simulink model "PMSM_ADRC_position_V21"  (R2024b)
settings: Solver=ode3  StartTime=0.0  StopTime=0.5  FixedStep=1e-6  RelTol=1e-3
model workspace (MAT data in the model file):
  PWM_Frequency = Simulink.Parameter
  PWM_Frequency.Value = 72000
  PWM_Frequency.Complexity = 'real'
  PWM_Frequency.Dimensions = [1 1]
  PWM_Frequency.DataType = 'double'
  TimerPeriod = 0.1
  Vdc = 12
  b0_id = 1333.33333333
  b0_iq = 1000
  b0_pos = 500
  idiq_ctrl_freq = 8000
  kd_pos = 200
  kp_id = 800
  kp_iq = 800
  kp_pos = 10000
  pos_ctrl_freq = 2000
  wc_pos = 50
  wo_id = 2000
  wo_iq = 2000
  wo_pos = 1000
undefined symbols (not defined in the file): Down, Up
libraries: eePwmGenerator x5, spsDCVoltageSourceLib x1, spsPermanentMagnetSynchronousMachineLib x1, spsUniversalBridgeLib x1, spspowerguiLib x1
settings Model: ParameterArgumentNames=wc_pos  Creator=shish  LastModifiedBy=HZSK

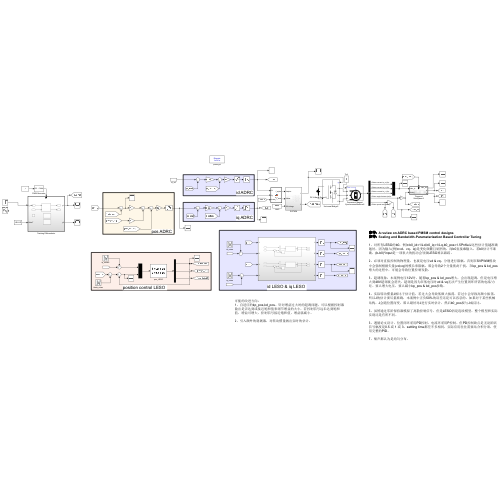
[thumbnail: Simulink's stored preview of the top-level diagram]
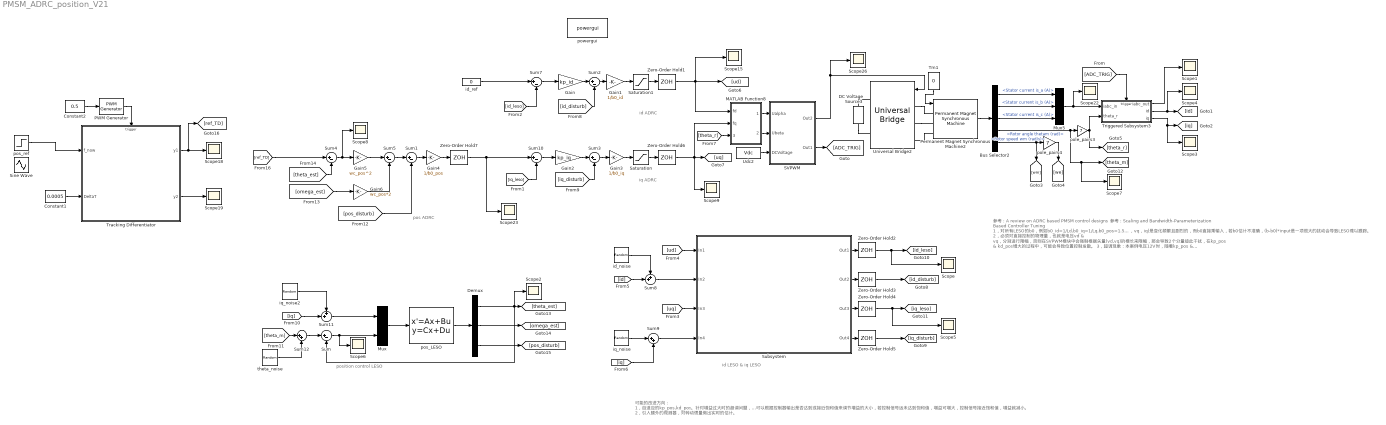
== system PMSM_ADRC_position_V21 ==
  note: 可能的改进方向：
      | 1，自适应的kp_pos,kd_pos。针对增益过大时的超调问题，可以根据控制器输出是否达到或接近饱和值来调节增益的大小，若控制信号远未达到饱和值，增益可增大，控制信号接近饱和值，增益就减小。
      |
      | 2，引入额外的观测器，对转动惯量做出实时的估计。
  note: id LESO & iq LESO
  note: 参考：A review on ADRC based PMSM control designs
      | 参考：Scaling and Bandwidth-Parameterization Based Controller Tuning
      |
      | 1，对所有LESO的b0，例如b0_id=1/Ld,b0_iq=1/Lq,b0_pos=1.5PnKe/J这些估计值越准确越好，因为输入(例如vd，vq，iq)是变化频繁且剧烈的，而b0直接乘输入，若b0估计不准确，(b-b0)*input是一项很大的扰动会导致LESO难以跟踪。
      |
      | 2，必须对直接控制的物理量，也就是电压vd & vq，分别进行限幅，否则在SVPWM模块中会强制根据矢量(vd,vq)的模长来限幅，那会导致2个分量彼此干扰，在kp_pos & kd_pos增大的过程中，可能会导致位置控制发散。
      |
      | 3，超调现象：本案例电压12V时，随着kp_pos & kd_pos增大，会出现超调，但是电压增大到48V超调就会消失。超调是因为在低电压时vd & vq无法产生位置闭环所需的电流/力矩。要么增大电压，要么减小kp_pos & kd_pos参数。
      |
      | 4，实际转动惯量J相比于估计值，若过大会导致低频大振荡，若过小会导致高频小振荡。所以J的估计要尽量准确，本案例中正负50%的误差还是可以容忍的。如果对于某些机械结构，J会随位置而变，那么最好对J进行实时估计，然后b0_pos要与J成反比。
      |
      | 5，虽然通过零阶保持器模拟了离散控制信号，但是LESO仍是连续模型，整个模型和实际实现还是有所不同。
      |
      | 6，遵循论文设计，位置闭环采用PD控制，电流环采用P控制。但PD控制缺点是无论阶跃信号幅度是0.5 或 1 或 3，settling time都差不多相同，实际应用往往需要结合积分项，使用完整的PID。
      |
      | 7，噪声都认为是均匀分布。
  note: position control LESO
  note: pos ADRC
  note: iq ADRC
  note: id ADRC
  Bus Selector2 : BusSelector  OutputSignals=Stator current is_a (A),Stator current is_b (A),Stator current is_c (A),Rotor angle thetam (rad),Rotor speed wm (rad/s)
  Constant1 : Constant  Value=0.0005
  Constant2 : Constant  Value=0.5
  DC Voltage Source3 : spsDCVoltageSourceLib/DC Voltage Source  Amplitude=Vdc  Measurements=Voltage
  Demux : Demux  Outputs=3
  Gain : Gain  Gain=kp_id
  Gain1 : Gain  Gain=1/b0_id
  Gain2 : Gain  Gain=kp_iq
  Gain3 : Gain  Gain=1/b0_iq
  Gain4 : Gain  Gain=1/b0_pos
  Gain5 : Gain  Gain=wc_pos^2
  Gain6 : Gain  Gain=wc_pos*2
  MATLAB Function8 : MATLAB Function  TreatAsAtomicUnit=on
  Mux : Mux  Inputs=2
  Mux5 : Mux  Inputs=3
  PWM Generator : eePwmGenerator/PWM Generator  CarrCount=Up  Tper=0.0005  Tdelay=0  Ts=5e-5
  Permanent Magnet Synchronous Machine2 : spsPermanentMagnetSynchronousMachineLib/Permanent Magnet Synchronous Machine  NbPhases=3  FluxDistribution=Sinusoidal  RotorType=Salient-pole  MechanicalLoad=Torque Tm  PresetModel=No  ShowDetailedParameters=on  MeasurementBus=off  Resistance=3  Inductance=8.5e-3  dqInductances=[0.75e-3,1.0e-3]  La=0.000395  MachineConstant=Flux linkage established by magnets (V.s)  Flux=0.0012  VoltageCst=1.5236  TorqueCst=0.0126  Flat=120  Mechanical=[1.2e-5 5e-6 7 0]  PolePairs=4  InitialConditions=[0,0, 0,0]  InitialConditions5ph=[0 0 0 0 0 0]  RefAngle=Aligned with phase A axis (original Park)  IterativeDiscreteModel=Trapezoidal non iterative  TsBlock=-1  TsPowergui=0
  SVPWM : Subsystem
  Saturation : Saturate  UpperLimit=2*Vdc/3  LowerLimit=-2*Vdc/3
  Saturation1 : Saturate  UpperLimit=2*Vdc/3  LowerLimit=-2*Vdc/3
  Scope{,1..9,15,18..19,22..23,26} (16 alike) : Scope
  Sine Wave : Sin  Amplitude=2  Frequency=2*pi  SampleTime=0
  Subsystem : Subsystem
  Sum{,1..5,7,10} (8 alike) : Sum  Inputs=|+-
  Sum11 : Sum  Inputs=++|
  Sum12 : Sum  Inputs=|++
  Sum8 : Sum  Inputs=++|
  Sum9 : Sum  Inputs=|++
  Tm1 : Constant  Value=0
  Tracking Differentiator : Subsystem
  Triggered Subsystem3 : Subsystem  TreatAsAtomicUnit=on
  Udc2 : Constant  Value=Vdc
  Universal Bridge2 : spsUniversalBridgeLib/Universal Bridge  Arms=3  SnubberResistance=1e5  SnubberCapacitance=inf  Device=MOSFET / Diodes  Ron=1e-3  Lon=0  ForwardVoltages="[  0  0  ]"  ForwardVoltage=0  GTOparameters=[ 10e-6 , 20e-6 ]  IGBTparameters=[ 1e-6 , 2e-6 ]  Measurements=None  Measurements_2=None  converterType=Rectifier
  Zero-Order Hold{1..6} (6 alike) : ZeroOrderHold  SampleTime=1.0/idiq_ctrl_freq
  Zero-Order Hold7 : ZeroOrderHold  SampleTime=1.0/pos_ctrl_freq
  id_noise : UniformRandomNumber  Minimum=-0.005  Maximum=0.005  SampleTime=1.0/40000
  id_ref : Constant  Value=0
  iq_noise : UniformRandomNumber  Minimum=-0.005  Maximum=0.005  SampleTime=1.0/40000
  iq_noise2 : UniformRandomNumber  Minimum=-0.005  Maximum=0.005  SampleTime=1.0/40000
  pole_pairs3 : Gain  Gain=7
  pole_pairs4 : Gain  Gain=7
  pos_LESO : StateSpace  A=[0 1 0; 0 0 1; 0 0 0]  B=[0 3*wo_pos;b0_pos 3*wo_pos^2;0 wo_pos^3]  C=[1 0 0;0 1 0;0 0 1]  D=[0 0;0 0;0 0]  InitialCondition=0
  pos_ref : Step  Time=0.1  After=3.0  SampleTime=0
  powergui : spspowerguiLib/powergui  Priority=1  SimulationMode=Discrete  SampleTime=1e-6  frequency=60  Iterations=50  frequencyindice=0  Pbase=100e6  ErrMax=1e-4  UnitsV=kV  UnitsW=MW  buscounter=0  FunctionMessages=off  echomessages=off  EnableUseOfTLC=off  CurrentSourceSwitches=off  DisableSnubberDevices=off  DisableRonSwitches=off  DisableVfSwitches=off  DisplayEquations=off  AutomaticDiscreteSolvers=off  SolverType=Tustin/Backward Euler (TBE)  Interpol=off  ExternalGateDelay=off  methode=off  Ts=100  x0status=blocks  SPID=on  SwTol=0  HookPort=off  NonlinearTolerance=1e-4  nMaxIteration=100  ContinueOnMaxIteration=off  RestoreLinks=warning  ResistiveCurrentMeasurement=off  Frange=[0:2:500]  Ylog=off  Xlog=on  ShowGrid=off  save=off  variable=ZData  structure=0  ZoomFFT=off  StartTime=0.0  cycles=1  DisplayStyle=1  fundamental=60  FreqAxis=off  MaxFrequency=1000  frequencyindicesteady=1  RmsSteady=1  display=off
  theta_noise : UniformRandomNumber  Minimum=-0.5*2*pi/4096  Maximum=0.5*2*pi/4096  SampleTime=1.0/2000
  wires:
  Bus Selector2/5 -> pole_pairs4/1, [wm]  "<Rotor speed wm (rad/s)>"
  MATLAB Function8/2(f_beta) -> SVPWM/2(Ubeta)
  Bus Selector2/3 -> Mux5/3  "<Stator current is_c (A)>"
  MATLAB Function8/1(f_alpha) -> SVPWM/1(Ualpha)
  Permanent Magnet Synchronous Machine2/1 -> Bus Selector2/1
  Bus Selector2/4 -> Scope7/1, [theta_m], pole_pairs3/1  "<Rotor angle thetam (rad)>"
  Udc2/1 -> SVPWM/3(DCVoltage)
  Bus Selector2/2 -> Mux5/2  "<Stator current is_b (A)>"
  Mux5/1 -> Triggered Subsystem3/1(iabc_in), Scope22/1
  Tm1/1 -> Permanent Magnet Synchronous Machine2/1
  SVPWM/1(Out2) -> Scope26/1, Universal Bridge2/1
  Bus Selector2/1 -> Mux5/1  "<Stator current is_a (A)>"
  Triggered Subsystem3/2(id) -> [id], Scope4/1
  Triggered Subsystem3/3(iq) -> [iq], Scope3/1
  pole_pairs4/1 -> [we]
  SVPWM/2(Out1) -> [ADC_TRIG]
  [ADC_TRIG] -> Triggered Subsystem3/Trigger
  pole_pairs3/1 -> Triggered Subsystem3/2(theta_r), [theta_r]
  [theta_r] -> MATLAB Function8/3(theta_r)
  Triggered Subsystem3/1(iabc_out) -> Scope1/1
  Subsystem/1(Out1) -> Zero-Order Hold2/1
  Subsystem/3(Out3) -> Zero-Order Hold4/1
  [ud] -> Subsystem/1(In1)
  [uq] -> Subsystem/3(In3)
  Subsystem/4(Out4) -> Zero-Order Hold5/1
  Mux/1 -> pos_LESO/1
  Sum/1 -> Scope6/1, Mux/2
  pos_LESO/1 -> Demux/1
  [pos_disturb] -> Sum1/2
  Sum1/1 -> Gain4/1
  Sum4/1 -> Scope8/1, Gain5/1
  Gain5/1 -> Sum5/1
  Gain6/1 -> Sum5/2
  Sum5/1 -> Sum1/1
  [theta_est] -> Sum4/2
  Gain4/1 -> Zero-Order Hold7/1
  Constant1/1 -> Tracking Differentiator/2(DeltaT)
  Tracking Differentiator/1(y1) -> [ref_TD], Scope18/1
  Constant2/1 -> PWM Generator/1
  PWM Generator/1 -> Tracking Differentiator/Trigger
  Tracking Differentiator/2(y2) -> Scope19/1
  [ref_TD] -> Sum4/1
  [omega_est] -> Gain6/1
  [id] -> Sum8/2
  [iq] -> Sum9/2
  id_noise/1 -> Sum8/1
  Sum8/1 -> Subsystem/2(In2)
  iq_noise/1 -> Sum9/1
  Sum9/1 -> Subsystem/4(In4)
  [iq] -> Sum11/2
  Sum11/1 -> Mux/1
  Sum12/1 -> Sum/1
  [theta_m] -> Sum12/1
  theta_noise/1 -> Sum12/2
  iq_noise2/1 -> Sum11/1
  Saturation1/1 -> Zero-Order Hold1/1
  Sum3/1 -> Gain3/1
  Sum10/1 -> Gain2/1
  Zero-Order Hold7/1 -> Scope23/1, Sum10/1
  Gain3/1 -> Saturation/1
  Gain2/1 -> Sum3/1
  [iq_disturb] -> Sum3/2
  [iq_leso] -> Sum10/2
  Sum7/1 -> Gain/1
  [id_disturb] -> Sum2/2
  Gain/1 -> Sum2/1
  id_ref/1 -> Sum7/1
  Gain1/1 -> Saturation1/1
  Sum2/1 -> Gain1/1
  [id_leso] -> Sum7/2
  Saturation/1 -> Zero-Order Hold6/1
  Zero-Order Hold6/1 -> Scope9/1, MATLAB Function8/2(fq), [uq]
  Zero-Order Hold1/1 -> Scope15/1, [ud], MATLAB Function8/1(fd)
  Zero-Order Hold3/1 -> [id_disturb]
  Subsystem/2(Out2) -> Zero-Order Hold3/1
  Zero-Order Hold4/1 -> Scope5/1, [iq_leso]
  Zero-Order Hold2/1 -> [id_leso], Scope/1
  Zero-Order Hold5/1 -> [iq_disturb]
  Demux/1 -> Sum/2, Scope2/1, [theta_est]
  Demux/2 -> [omega_est]
  Demux/3 -> [pos_disturb]
  pos_ref/1 -> Tracking Differentiator/1(f_now)
  connections:
  Universal Bridge2/LConn2 -- Permanent Magnet Synchronous Machine2/LConn2
  Universal Bridge2/LConn1 -- Permanent Magnet Synchronous Machine2/LConn1
  DC Voltage Source3/LConn1 -- Universal Bridge2/RConn2
  DC Voltage Source3/RConn1 -- Universal Bridge2/RConn1
  Universal Bridge2/LConn3 -- Permanent Magnet Synchronous Machine2/LConn3

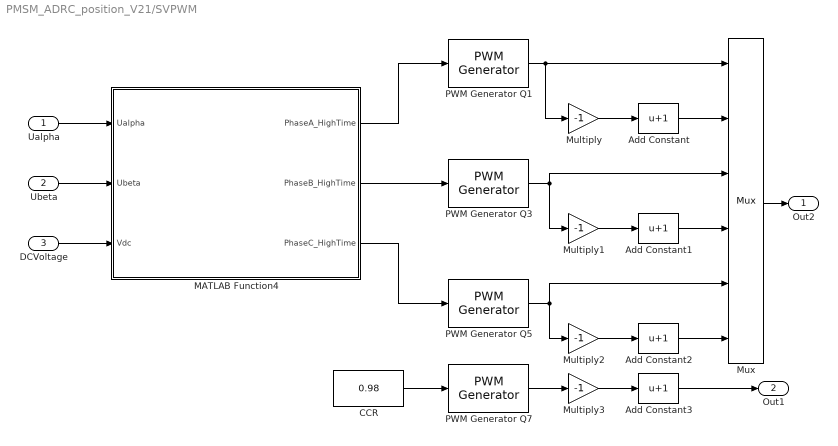
== system PMSM_ADRC_position_V21/SVPWM ==
  Ualpha : Inport
  Ubeta : Inport  Port=2
  DCVoltage : Inport  Port=3
  Add Constant{,1..3} (4 alike) : Bias  Bias=1  SaturateOnIntegerOverflow=off
  CCR : Constant  Value=0.98
  MATLAB Function4 : MATLAB Function  TreatAsAtomicUnit=on
  Multiply{,1..3} (4 alike) : Gain  Gain=-1
  Mux : Mux  Inputs=6
  PWM Generator Q{1,3,5,7} (4 alike) : eePwmGenerator/PWM Generator  CarrCount=Up-Down  Tper=1.0/PWM_Frequency  Tdelay=0  Ts=1E-6
  Out2 : Outport
  Out1 : Outport  Port=2
  wires:
  PWM Generator Q5/1 -> Mux/5, Multiply2/1
  PWM Generator Q1/1 -> Multiply/1, Mux/1
  Add Constant1/1 -> Mux/4
  Ubeta/1 -> MATLAB Function4/2(Ubeta)
  DCVoltage/1 -> MATLAB Function4/3(Vdc)
  MATLAB Function4/3(PhaseC_HighTime) -> PWM Generator Q5/1
  Multiply/1 -> Add Constant/1
  Multiply2/1 -> Add Constant2/1
  Add Constant/1 -> Mux/2
  MATLAB Function4/2(PhaseB_HighTime) -> PWM Generator Q3/1
  Add Constant2/1 -> Mux/6
  Multiply1/1 -> Add Constant1/1
  MATLAB Function4/1(PhaseA_HighTime) -> PWM Generator Q1/1
  Ualpha/1 -> MATLAB Function4/1(Ualpha)
  PWM Generator Q3/1 -> Mux/3, Multiply1/1
  PWM Generator Q7/1 -> Multiply3/1
  CCR/1 -> PWM Generator Q7/1
  Multiply3/1 -> Add Constant3/1
  Add Constant3/1 -> Out1/1
  Mux/1 -> Out2/1

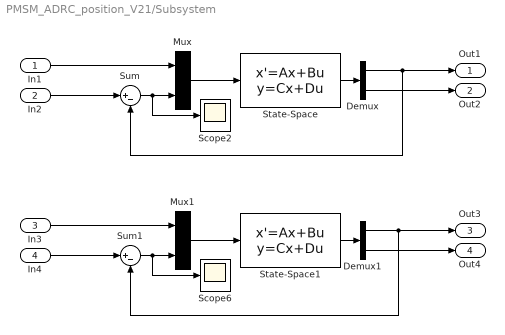
== system PMSM_ADRC_position_V21/Subsystem ==
  In1 : Inport
  In2 : Inport  Port=2
  In3 : Inport  Port=3
  In4 : Inport  Port=4
  Demux : Demux  Outputs=2
  Demux1 : Demux  Outputs=2
  Mux : Mux  Inputs=2
  Mux1 : Mux  Inputs=2
  Scope2 : Scope
  Scope6 : Scope
  State-Space : StateSpace  A=[0 1;0 0]  B=[b0_id 2*wo_id;0 wo_id^2]  C=[1 0;0 1]  D=[0 0;0 0]  InitialCondition=0
  State-Space1 : StateSpace  A=[0 1;0 0]  B=[b0_iq 2*wo_iq;0 wo_iq^2]  C=[1 0;0 1]  D=[0 0; 0 0]  InitialCondition=0
  Sum : Sum  Inputs=|+-
  Sum1 : Sum  Inputs=|+-
  Out1 : Outport
  Out2 : Outport  Port=2
  Out3 : Outport  Port=3
  Out4 : Outport  Port=4
  wires:
  Demux1/2 -> Out4/1
  Sum/1 -> Scope2/1, Mux/2
  Demux1/1 -> Out3/1, Sum1/2
  Sum1/1 -> Scope6/1, Mux1/2
  In1/1 -> Mux/1
  State-Space/1 -> Demux/1
  Mux/1 -> State-Space/1
  State-Space1/1 -> Demux1/1
  Mux1/1 -> State-Space1/1
  In4/1 -> Sum1/1
  In2/1 -> Sum/1
  In3/1 -> Mux1/1
  Demux/1 -> Out1/1, Sum/2
  Demux/2 -> Out2/1

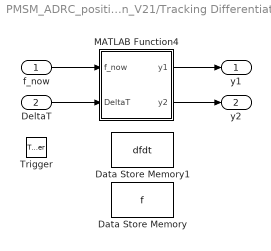
== system PMSM_ADRC_position_V21/Tracking Differentiator ==
  f_now : Inport
  DeltaT : Inport  Port=2
  Trigger : TriggerPort  VariantControl=(inherit)  PortDimensions=1
  Data Store Memory : DataStoreMemory  DataStoreName=f  WriteAfterWriteMsg=warning  ShowAdditionalParam=off  OutDataTypeStr=double
  Data Store Memory1 : DataStoreMemory  DataStoreName=dfdt  WriteAfterWriteMsg=warning  ShowAdditionalParam=off  OutDataTypeStr=double
  MATLAB Function4 : MATLAB Function  TreatAsAtomicUnit=on
  y1 : Outport
  y2 : Outport  Port=2
  wires:
  f_now/1 -> MATLAB Function4/1(f_now)
  DeltaT/1 -> MATLAB Function4/2(DeltaT)
  MATLAB Function4/1(y1) -> y1/1
  MATLAB Function4/2(y2) -> y2/1

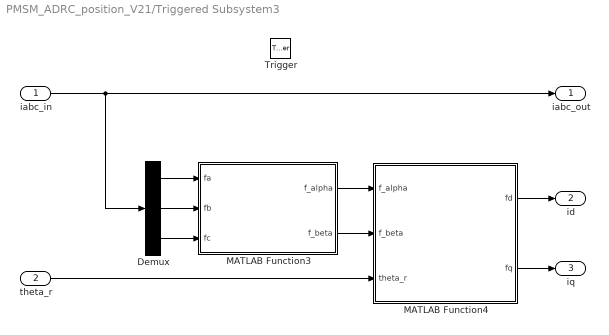
== system PMSM_ADRC_position_V21/Triggered Subsystem3 ==
  iabc_in : Inport
  theta_r : Inport  Port=2
  Trigger : TriggerPort  VariantControl=(inherit)
  Demux : Demux  Outputs=3
  MATLAB Function3 : MATLAB Function  TreatAsAtomicUnit=on
  MATLAB Function4 : MATLAB Function  TreatAsAtomicUnit=on
  iabc_out : Outport
  id : Outport  Port=2
  iq : Outport  Port=3
  wires:
  iabc_in/1 -> Demux/1, iabc_out/1
  Demux/3 -> MATLAB Function3/3(fc)
  Demux/2 -> MATLAB Function3/2(fb)
  Demux/1 -> MATLAB Function3/1(fa)
  MATLAB Function3/1(f_alpha) -> MATLAB Function4/1(f_alpha)
  MATLAB Function3/2(f_beta) -> MATLAB Function4/2(f_beta)
  theta_r/1 -> MATLAB Function4/3(theta_r)
  MATLAB Function4/1(fd) -> id/1
  MATLAB Function4/2(fq) -> iq/1

== matlab function PMSM_ADRC_position_V21/Tracking Differentiator/MATLAB Function4 ==
  data: f_now input; y1 output; f data_store_memory; dfdt data_store_memory; DeltaT input; y2 output
function [y1,y2]= TD(f_now, DeltaT)
	global f;
    global dfdt;

	x1k = f;
	x2k = dfdt;

	factor = x2k*x2k/1000.0;
    if factor < 1.0
		factor = 1.0;
    end
    h = DeltaT;
	h0 = 2*h;
    r = 50/h;
	fh = fhan(x1k - f_now, x2k, r*factor, h0);
	
	
	x1k = x1k + h*x2k;
	x2k = x2k + h*fh;

	f = x1k;
	dfdt = x2k;
	
	y1 = x1k;
    y2 = x2k;

end



function y = fsg(x,d)
 y = (sign(x+d) - sign(x-d))/2.0;
end



function y = fhan(x1,x2,r,h)
 	d = r*h*h;
	a0 = h*x2;
	y = x1 + a0;

	a1 = sqrt(d*(d+8*abs(y)));
	a2 = a0 + 0.5*sign(y)*(a1-d);

	temp1 = fsg(y,d);
	a = (a0+y)*temp1 + a2*(1-temp1);

	temp2 = fsg(a,d);
	ret = -r*((a/d)*temp2 + sign(a)*(1-temp2));
	y = ret;
end

== matlab function PMSM_ADRC_position_V21/MATLAB Function8 ==
  data: fd input; f_alpha output; fq input; theta_r input; f_beta output
function [f_alpha,f_beta]= fcn(fd,fq,theta_r)
c = cos(theta_r);
s = sin(theta_r);
f_alpha =  c*fd - s*fq;
f_beta =  s*fd + c*fq;

== matlab function PMSM_ADRC_position_V21/SVPWM/MATLAB Function4 ==
  data: Ualpha input; PhaseA_HighTime output; Ubeta input; Vdc input; PhaseB_HighTime output; PhaseC_HighTime output
function [PhaseA_HighTime,PhaseB_HighTime,PhaseC_HighTime] = SVPWM_calculate(Ualpha,Ubeta,Vdc)

% unit:V %

%step 1,which sector?%
if Ualpha >= 0
    %sector=1,2,5,6%
    if Ubeta >= 0
        %sector=1,2%
        if Ubeta > sqrt(3)*Ualpha
            sector=2;
        else
            sector=1;
        end
    else
        %sector=5,6%
        if -Ubeta > sqrt(3)*Ualpha
            sector=5;
        else
            sector=6;
        end
    end
else
    %sector=2,3,4,5%
    if Ubeta >= 0
        %sector=2,3%
        if Ubeta > -sqrt(3)*Ualpha
            sector=2;
        else
            sector=3;
        end
    else
        %sector=4,5%
        if -Ubeta > -sqrt(3)*Ualpha
            sector=5;
        else
            sector=4;
        end
    end
end

%step 2,vector decompose%
v1 = (2*Vdc/3)*[ 1,0];
v2 = (2*Vdc/3)*[ 0.5, 0.5*sqrt(3)];
v3 = (2*Vdc/3)*[-0.5, 0.5*sqrt(3)];
v4 = (2*Vdc/3)*[-1,0];
v5 = (2*Vdc/3)*[-0.5,-0.5*sqrt(3)];
v6 = (2*Vdc/3)*[ 0.5,-0.5*sqrt(3)];

if sector == 1
    vm=v1;vn=v2;
elseif sector == 2
    vm=v2;vn=v3;
elseif sector == 3
    vm=v3;vn=v4;
elseif sector == 4
    vm=v4;vn=v5;
elseif sector == 5
    vm=v5;vn=v6;
else
    vm=v6;vn=v1;
end

cm = (Ualpha*vn(2) - Ubeta*vn(1))/(vm(1)*vn(2) - vm(2)*vn(1));

if abs(vn(1))>1e-7
    cn = (Ualpha-cm*vm(1))/vn(1);
else
    cn = (Ubeta-cm*vm(2))/vn(2);
end
c_summ = cm+cn;
% if c_summ > 1
%     cm = cm/c_summ;
%     cn = cn/c_summ;
% end
if c_summ > 0.95
    cm = 0.95*cm/c_summ;
    cn = 0.95*cn/c_summ;
end

c0 = (1-cm-cn);
c0 = 0.5*c0;
c7 = c0;

%step 3,duty cycle%
if sector == 1
    %v1:100  v2:110%
    PhaseA_HighTime = cm+cn+c7;
    PhaseB_HighTime = cn+c7;
    PhaseC_HighTime = c7;
elseif sector == 2
    %v2:110  v3:010%
    PhaseA_HighTime = cm+c7;
    PhaseB_HighTime = cm+cn+c7;
    PhaseC_HighTime = c7;
elseif sector == 3
    %v3:010  v4:011%
    PhaseA_HighTime = c7;
    PhaseB_HighTime = cm+cn+c7;
    PhaseC_HighTime = cn+c7;
elseif sector == 4
    %v4:011  v5:001%
    PhaseA_HighTime = c7;
    PhaseB_HighTime = cm+c7;
    PhaseC_HighTime = cm+cn+c7;
elseif sector == 5
    %v5:001  v6:101%
    PhaseA_HighTime = cn+c7;
    PhaseB_HighTime = c7;
    PhaseC_HighTime = cm+cn+c7;
else
    %v6:101  v1:100%
    PhaseA_HighTime = cm+cn+c7;
    PhaseB_HighTime = c7;
    PhaseC_HighTime = cm+c7;
end

== matlab function PMSM_ADRC_position_V21/Triggered Subsystem3/MATLAB Function3 ==
  data: fa input; f_alpha output; fb input; fc input; f_beta output
function [f_alpha,f_beta]= ABC_to_AlphaBeta(fa,fb,fc)
f_alpha = (2/3)*(fa-0.5*(fb+fc));
f_beta = (2/3)*(0.5*sqrt(3)*(fb-fc));

== matlab function PMSM_ADRC_position_V21/Triggered Subsystem3/MATLAB Function4 ==
  data: f_alpha input; fd output; f_beta input; fq output; theta_r input
function [fd,fq]= AlphaBeta_to_dq(f_alpha,f_beta,theta_r)

c = cos(theta_r);
s = sin(theta_r);
fd =  c*f_alpha + s*f_beta;
fq = -s*f_alpha + c*f_beta;
